simulink model "sampleModel1948_2_sub_sub_sub"  (R2023a)
settings: Solver=VariableStepAuto  StartTime=0.0  StopTime=10.0  RelTol=1e-3
libraries: simulink x3, hdlsllib x3
settings Model: Creator=user1  LastModifiedBy=user1

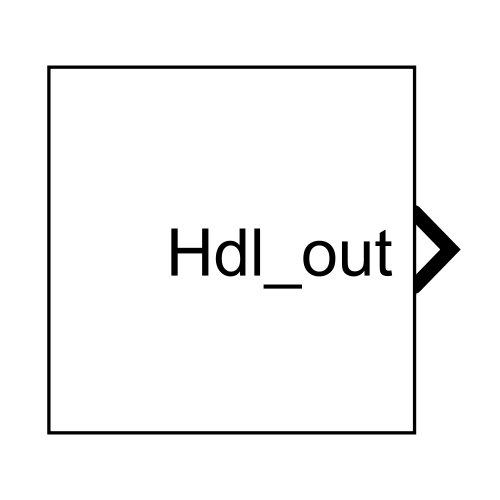
[thumbnail: Simulink's stored preview of the top-level diagram]
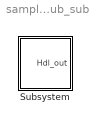
== system sampleModel1948_2_sub_sub_sub ==
  Subsystem : Subsystem

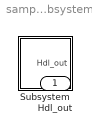
== system sampleModel1948_2_sub_sub_sub/Subsystem ==
  Subsystem : Subsystem
  Hdl_out : Outport  OutDataTypeStr=uint8

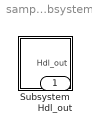
== system sampleModel1948_2_sub_sub_sub/Subsystem/Subsystem ==
  Subsystem : Subsystem
  Hdl_out : Outport  OutDataTypeStr=uint8

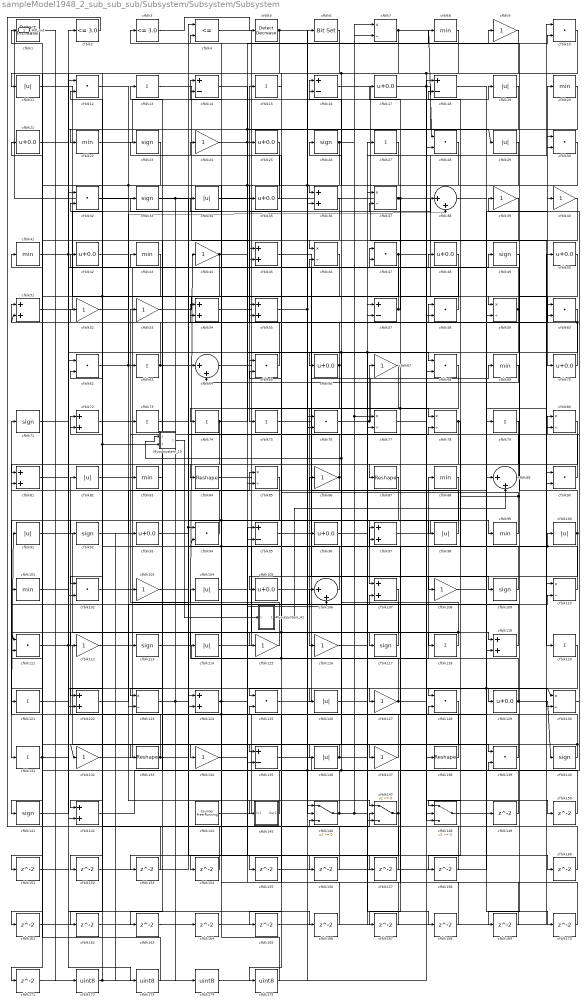
== system sampleModel1948_2_sub_sub_sub/Subsystem/Subsystem/Subsystem ==
  Mysubsystem_19 : Subsystem  TreatAsAtomicUnit=on  RTWFcnName=Mysubsystem_19
      settings: RTWFcnNameOpts=User specified  RTWFileNameOpts=Use function name
  Mysubsystem_41 : Subsystem  TreatAsAtomicUnit=on  RTWFcnName=Mysubsystem_41
      settings: RTWFcnNameOpts=User specified  RTWFileNameOpts=Use function name
  cfblk1 : simulink/Logic and Bit Operations/Detect Increase  vinit=0.0  OutDataTypeStr=uint8
      settings: LibrarySourceBlock=|
      | hdlsllib/Logic and Bit
      | Operations/Detect
      | Increase
  cfblk{10,12,28,30,32,47,58,60,62,65,68,76,90,94,102,111,125,128,139} (19 alike) : DotProduct  OutDataTypeStr=uint8
  cfblk{11,19,29,34,82,91,98,100,104,114,126,136} (12 alike) : Abs  OutDataTypeStr=uint8  SaturateOnIntegerOverflow=off
  cfblk{8,20,22,41,43,69,83,88,99,101} (10 alike) : MinMax  OutDataTypeStr=uint8
  cfblk{9,24,39..40,44,52..53,67,86,103,108,112,115..116,127,132,134,137} (18 alike) : Gain  OutDataTypeStr=uint8
  cfblk{17,21,25,35,42,48,50,66,70,93,96,105,129} (13 alike) : Bias  Bias=0.0  SaturateOnIntegerOverflow=off
  cfblk{38,64,89,106} (4 alike) : Sum  Inputs=|++  OutDataTypeStr=uint8
  cfblk{36,45,51,54..55,72,81,97,107,119,122,124,142} (13 alike) : Sum  OutDataTypeStr=uint8
  cfblk{23,26,33,49,71,92,109,113,117,140..141} (11 alike) : Signum
  cfblk{7,37,46,59,77..78,80,85,110,123,130} (11 alike) : Product  Inputs=*/  OutDataTypeStr=uint8  RndMeth=Zero  SaturateOnIntegerOverflow=on
  cfblk{13,15,27,63,73..75,79,118,120..121,131} (12 alike) : Sum  Inputs=+  OutDataTypeStr=uint8
  cfblk{84,87,133,138} (4 alike) : Reshape
  cfblk{14,16,18,57,95,135} (6 alike) : Sum  Inputs=+-  OutDataTypeStr=uint8
  cfblk144 : hdlsllib/Sources/Counter Free-Running  NumBits=16  tsamp=-1
  cfblk145 : Subsystem
      settings: LibrarySourceBlock=|
      | hdlsllib/Ports &
      | Subsystems/Subsystem
  cfblk146 : Switch  OutDataTypeStr=uint8  SaturateOnIntegerOverflow=off  InputSameDT=off
  cfblk147 : Switch  OutDataTypeStr=uint8  SaturateOnIntegerOverflow=off  InputSameDT=off
  cfblk148 : Switch  OutDataTypeStr=uint8  SaturateOnIntegerOverflow=off  InputSameDT=off
  cfblk{149..158,160..171} (22 alike) : Delay  SampleTime=1
  cfblk{172..175} (4 alike) : DataTypeConversion  OutDataTypeStr=uint8  SaturateOnIntegerOverflow=off  RndMeth=Floor
  cfblk2 : hdlsllib/Logic and Bit Operations/Compare To Constant  relop=<=  const=3.0  OutDataTypeStr=uint8
  cfblk3 : hdlsllib/Logic and Bit Operations/Compare To Constant  relop=<=  const=3.0  OutDataTypeStr=uint8
  cfblk4 : RelationalOperator  Operator=<=  OutDataTypeStr=boolean  InputSameDT=off
  cfblk5 : simulink/Logic and Bit Operations/Detect Decrease  vinit=0.0  OutDataTypeStr=uint8
      settings: LibrarySourceBlock=|
      | hdlsllib/Logic and Bit
      | Operations/Detect
      | Decrease
  cfblk6 : simulink/Logic and Bit Operations/Bit Set  iBit=0
      settings: LibrarySourceBlock=|
      | hdlsllib/Logic and Bit
      | Operations/Bit Set
  Hdl_out : Outport  OutDataTypeStr=uint8
  wires:
  cfblk91/1 -> cfblk117/1
  cfblk63/1 -> cfblk98/1, cfblk51/1
  cfblk113/1 -> cfblk88/1
  cfblk11/1 -> cfblk70/1
  cfblk127/1 -> cfblk30/1, cfblk55/2, cfblk44/1
  cfblk140/1 -> cfblk43/1, cfblk132/1
  cfblk97/1 -> cfblk99/1
  cfblk135/1 -> cfblk39/1
  cfblk4/1 -> cfblk119/1
  cfblk138/1 -> cfblk82/1
  cfblk125/1 -> cfblk49/1
  cfblk70/1 -> cfblk20/1
  cfblk30/1 -> cfblk75/1
  cfblk112/1 -> cfblk47/1
  cfblk115/1 -> cfblk53/1
  cfblk90/1 -> cfblk63/1
  cfblk16/1 -> cfblk120/1
  cfblk65/1 -> cfblk15/1
  cfblk79/1 -> cfblk148/1
  cfblk111/1 -> cfblk124/2, cfblk139/1
  cfblk108/1 -> cfblk79/1
  cfblk54/1 -> cfblk68/1
  cfblk142/1 -> cfblk96/1, cfblk57/1
  cfblk110/1 -> cfblk100/1, cfblk35/1
  cfblk45/1 -> cfblk108/1
  cfblk99/1 -> cfblk18/2, cfblk25/1
  cfblk100/1 -> cfblk165/1, cfblk3/1
  cfblk68/1 -> cfblk167/1, cfblk85/2
  cfblk40/1 -> cfblk46/1
  cfblk13/1 -> cfblk65/1
  cfblk66/1 -> cfblk54/1, cfblk74/1
  cfblk22/1 -> cfblk19/1
  cfblk114/1 -> cfblk50/1
  cfblk1/1 -> cfblk172/1
  cfblk64/1 -> cfblk116/1
  cfblk52/1 -> cfblk103/1
  cfblk133/1 -> cfblk97/1, cfblk71/1
  cfblk87/1 -> cfblk131/1
  cfblk28/1 -> cfblk36/2, cfblk123/2, cfblk92/1
  cfblk85/1 -> cfblk154/1, cfblk102/1
  cfblk77/1 -> cfblk138/1
  cfblk43/1 -> cfblk171/1, cfblk142/1
  cfblk62/1 -> cfblk38/2, cfblk127/1
  cfblk101/1 -> cfblk62/1
  cfblk20/1 -> cfblk22/1
  cfblk71/1 -> cfblk32/1
  cfblk81/1 -> cfblk47/2
  cfblk57/1 -> cfblk17/1, cfblk34/1
  cfblk95/1 -> cfblk69/1
  cfblk80/1 -> cfblk122/1
  cfblk24/1 -> cfblk10/2, cfblk68/2
  cfblk33/1 -> cfblk164/1, cfblk147/1
  cfblk15/1 -> cfblk45/1
  cfblk21/1 -> cfblk66/1
  cfblk2/1 -> cfblk147/2
  cfblk132/1 -> cfblk4/1
  cfblk116/1 -> cfblk58/1
  cfblk49/1 -> cfblk129/1
  cfblk126/1 -> cfblk128/1
  cfblk146/1 -> cfblk12/2, cfblk27/1, cfblk77/1, cfblk7/2
  cfblk7/1 -> cfblk28/1, cfblk36/1, cfblk142/2
  cfblk139/1 -> cfblk86/1
  cfblk9/1 -> cfblk112/1
  cfblk48/1 -> cfblk137/1
  cfblk17/1 -> cfblk130/2, cfblk89/1
  cfblk8/1 -> cfblk28/2, cfblk141/1
  cfblk141/1 -> cfblk45/2
  cfblk55/1 -> cfblk109/1, cfblk9/1
  cfblk26/1 -> cfblk7/1, cfblk125/1
  cfblk137/1 -> cfblk91/1, cfblk24/1, cfblk94/2
  cfblk130/1 -> cfblk80/1
  cfblk37/1 -> Hdl_out/1, cfblk87/1, cfblk90/1
  cfblk117/1 -> Mysubsystem_19/1(In1), cfblk42/1
  cfblk86/1 -> cfblk81/2, cfblk65/2
  cfblk53/1 -> cfblk59/1
  cfblk58/1 -> cfblk26/1
  cfblk67/1 -> cfblk146/2
  cfblk76/1 -> cfblk38/1, cfblk67/1
  cfblk19/1 -> cfblk122/2
  cfblk59/1 -> cfblk16/2, cfblk95/2
  cfblk124/1 -> cfblk106/2, cfblk14/1
  cfblk103/1 -> cfblk78/2, cfblk94/1
  cfblk119/1 -> cfblk101/1
  cfblk82/1 -> cfblk83/1
  cfblk118/1 -> cfblk46/2, cfblk111/1
  cfblk27/1 -> cfblk84/1
  cfblk78/1 -> cfblk158/1, cfblk105/1
  cfblk144/1 -> cfblk59/2
  cfblk46/1 -> cfblk123/1
  cfblk145/1(Out1) -> cfblk72/1
  cfblk131/1 -> cfblk41/1, cfblk128/2
  cfblk107/1 -> cfblk155/1, cfblk134/1
  cfblk123/1 -> cfblk174/1, cfblk157/1
  cfblk88/1 -> cfblk107/1
  cfblk105/1 -> cfblk40/1
  cfblk60/1 -> cfblk51/2, cfblk147/3, cfblk136/1, cfblk115/1
  cfblk74/1 -> cfblk37/2, cfblk121/1
  cfblk42/1 -> cfblk113/1
  cfblk44/1 -> cfblk8/1, cfblk133/1
  cfblk104/1 -> cfblk107/2
  cfblk29/1 -> cfblk152/1, cfblk135/2
  cfblk25/1 -> cfblk114/1
  cfblk14/1 -> cfblk76/2, cfblk29/1
  cfblk12/1 -> cfblk73/1
  cfblk121/1 -> cfblk12/1
  cfblk35/1 -> cfblk23/1
  cfblk10/1 -> cfblk11/1
  cfblk92/1 -> cfblk85/1
  cfblk34/1 -> cfblk78/1
  cfblk5/1 -> cfblk162/1, cfblk77/2
  cfblk94/1 -> cfblk21/1
  cfblk93/1 -> cfblk60/2
  cfblk109/1 -> cfblk48/1
  cfblk106/1 -> cfblk72/2, Mysubsystem_19/2(In2)
  cfblk98/1 -> cfblk16/1
  cfblk18/1 -> cfblk170/1, cfblk130/1
  cfblk72/1 -> cfblk126/1
  cfblk136/1 -> cfblk30/2, cfblk135/1
  cfblk38/1 -> cfblk80/2
  cfblk129/1 -> cfblk54/2, cfblk140/1
  cfblk120/1 -> cfblk148/2
  cfblk89/1 -> cfblk55/1
  cfblk147/1 -> cfblk163/1, cfblk13/1, cfblk106/1
  cfblk122/1 -> cfblk110/2
  cfblk84/1 -> cfblk148/3
  cfblk3/1 -> cfblk5/1
  cfblk102/1 -> cfblk145/1(In1)
  cfblk47/1 -> cfblk150/1, cfblk102/2
  cfblk83/1 -> cfblk33/1
  cfblk41/1 -> cfblk166/1, cfblk2/1
  cfblk51/1 -> cfblk10/1
  cfblk32/1 -> cfblk118/1
  cfblk69/1 -> cfblk64/2
  cfblk75/1 -> cfblk18/1
  cfblk36/1 -> cfblk81/1
  cfblk148/1 -> cfblk149/1
  cfblk149/1 -> cfblk139/2
  cfblk150/1 -> cfblk111/2
  cfblk128/1 -> cfblk151/1
  cfblk152/1 -> cfblk64/1
  cfblk39/1 -> cfblk153/1
  cfblk153/1 -> cfblk62/2
  cfblk154/1 -> cfblk124/1
  cfblk155/1 -> cfblk119/2
  cfblk134/1 -> cfblk156/1
  cfblk156/1 -> cfblk146/3
  cfblk157/1 -> cfblk14/2
  cfblk158/1 -> cfblk32/2
  cfblk73/1 -> cfblk160/1
  cfblk160/1 -> cfblk76/1
  cfblk23/1 -> cfblk161/1
  cfblk161/1 -> cfblk60/1
  cfblk162/1 -> cfblk110/1
  cfblk163/1 -> cfblk90/2
  cfblk164/1 -> cfblk57/2
  cfblk165/1 -> cfblk37/1
  cfblk166/1 -> cfblk125/2
  cfblk167/1 -> cfblk95/1
  cfblk96/1 -> cfblk168/1
  cfblk168/1 -> cfblk146/1
  cfblk50/1 -> cfblk169/1
  cfblk169/1 -> cfblk4/2
  cfblk170/1 -> cfblk97/2
  cfblk171/1 -> cfblk58/2
  cfblk172/1 -> cfblk93/1, cfblk52/1
  cfblk151/1 -> cfblk173/1
  cfblk173/1 -> cfblk1/1
  cfblk174/1 -> cfblk6/1
  cfblk6/1 -> cfblk175/1
  cfblk175/1 -> cfblk104/1
  Mysubsystem_19/1(Out1) -> Mysubsystem_41/1(In1)
  Mysubsystem_41/1(Out1) -> cfblk89/2

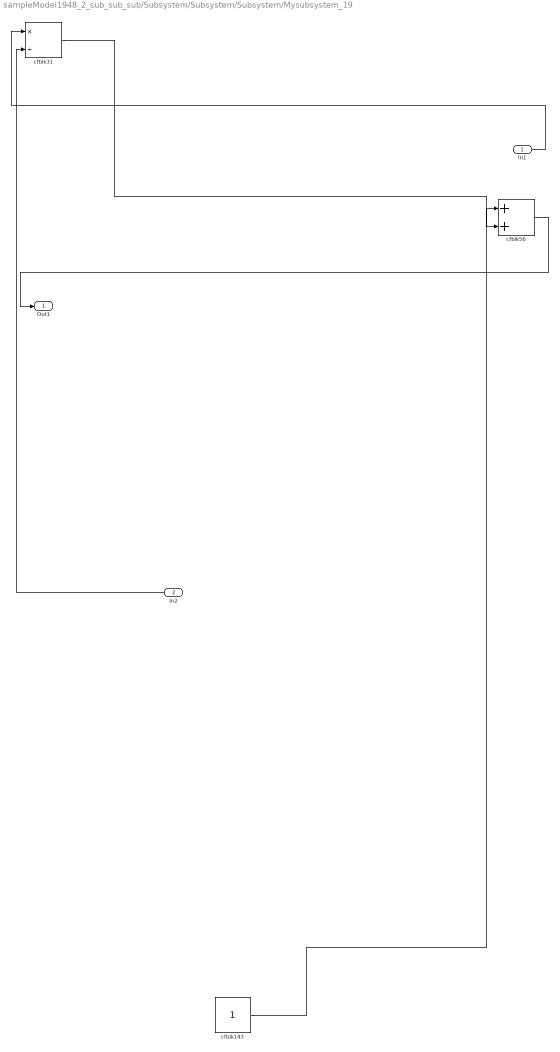
== system sampleModel1948_2_sub_sub_sub/Subsystem/Subsystem/Subsystem/Mysubsystem_19 ==
  In1 : Inport
  In2 : Inport  Port=2
  cfblk143 : Constant  SampleTime=-1
  cfblk31 : Product  Inputs=*/  RndMeth=Zero  SaturateOnIntegerOverflow=on
  cfblk56 : Sum
  Out1 : Outport
  wires:
  In1/1 -> cfblk31/1
  cfblk143/1 -> cfblk56/1
  cfblk31/1 -> cfblk56/2
  In2/1 -> cfblk31/2
  cfblk56/1 -> Out1/1

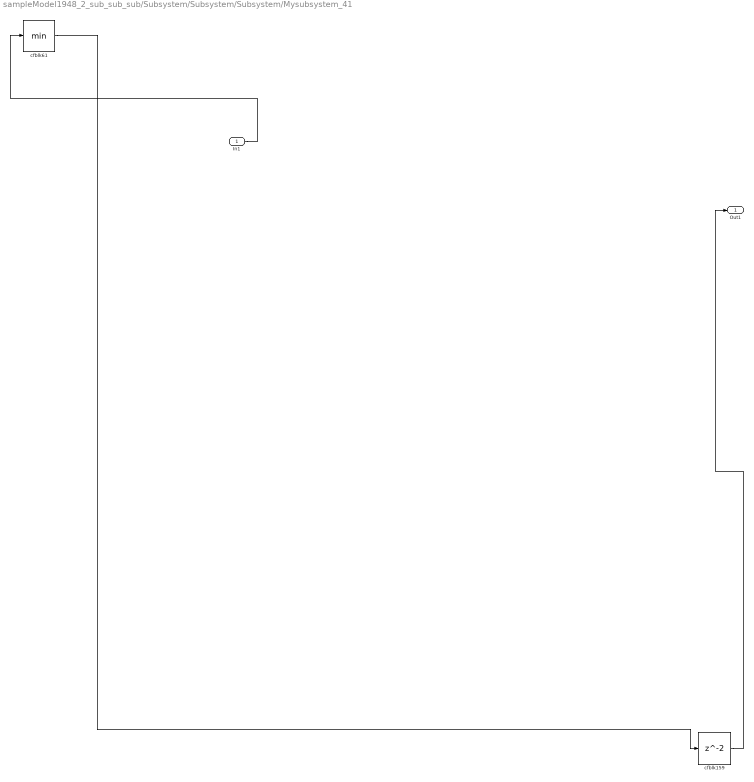
== system sampleModel1948_2_sub_sub_sub/Subsystem/Subsystem/Subsystem/Mysubsystem_41 ==
  In1 : Inport
  cfblk159 : Delay  SampleTime=1
  cfblk61 : MinMax
  Out1 : Outport
  wires:
  In1/1 -> cfblk61/1
  cfblk159/1 -> Out1/1
  cfblk61/1 -> cfblk159/1

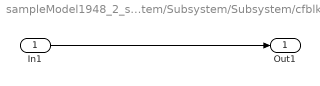
== system sampleModel1948_2_sub_sub_sub/Subsystem/Subsystem/Subsystem/cfblk145 ==
  In1 : Inport
  Out1 : Outport
  wires:
  In1/1 -> Out1/1
